simulink model "power_blk"  (R2019a)
settings: Solver=VariableStepAuto  StartTime=0.0  StopTime=10.0  RelTol=1e-3
libraries: xbsIndex_r4 x2
settings Model: Creator=mybur  LastModifiedBy=mybur

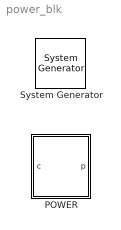
== system power_blk ==
  " System Generator" : xbsIndex_r4/ System Generator  Tag=genX  xilinxfamily=kintex7  part=xc7k325t  speed=-3  package=fbg676  synthesis_tool=Vivado  clock_wrapper=Clock Enables  directory=./netlist  proj_type=Vivado  Synth_file=Vivado Synthesis Defaults  Impl_file=Vivado Implementation Defaults  testbench=off  simulink_period=1  sysclk_period=10  dcm_input_clock_period=10  incr_netlist=off  trim_vbits=Everywhere in SubSystem  dbl_ovrd=According to Block Masks  core_generation=According to Block Masks  run_coregen=off  deprecated_control=off  eval_field=0  block_type=sysgen
  POWER : Subsystem  mask(Power){BitWidth=8, add_latency=0, mult_latency=0, use_dsp=on}
      mask prompts: BitWidth "Bit Width"; add_latency "Add Latency"; mult_latency "Mult Latency"; use_dsp "Use DSP48?"
      mask help: Squares real and imaginary components of complex input and adds them.
      mask init:
      | Simulink.Block.eval([gcb, '/power']);

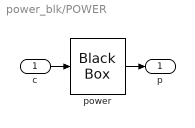
== system power_blk/POWER ==
  c : Inport
  power : xbsIndex_r4/Black Box  init_code=power_config  sim_method=ISE Simulator  verbose=off  block_type=blackbox2
  p : Outport
  wires:
  c/1 -> power/1
  power/1 -> p/1
